simulink model "Digital-Memory-Architecture"  (R2024b)
settings: Solver=VariableStepAuto  StartTime=0.0  StopTime=10.0  RelTol=1e-3
libraries: simulink_extras x129
(part 3 of 5)

== system Digital-Memory-Architecture/BitCell23 ==
  D : Inport
  WE : Inport  Port=2
  CLK : Inport  Port=3
  Constant : Constant
  D Flip-Flop : simulink_extras/Flip Flops/D Flip-Flop
  Logical Operator : Logic  Operator=NOT  IconShape=distinctive  AllPortsSameDT=off  OutDataTypeStr=boolean
  Logical Operator1 : Logic  IconShape=distinctive  AllPortsSameDT=off  OutDataTypeStr=boolean
  Logical Operator2 : Logic  IconShape=distinctive  AllPortsSameDT=off  OutDataTypeStr=boolean
  Logical Operator3 : Logic  Operator=OR  IconShape=distinctive  AllPortsSameDT=off  OutDataTypeStr=boolean
  Q : Outport
  wires:
  Logical Operator2/1 -> Logical Operator3/2
  CLK/1 -> D Flip-Flop/2
  Logical Operator1/1 -> Logical Operator3/1
  Constant/1 -> D Flip-Flop/3
  D Flip-Flop/1 -> Q/1, Logical Operator2/2
  Logical Operator3/1 -> D Flip-Flop/1
  Logical Operator/1 -> Logical Operator2/1
  WE/1 -> Logical Operator/1, Logical Operator1/2
  D/1 -> Logical Operator1/1

== system Digital-Memory-Architecture/BitCell24 ==
  D : Inport
  WE : Inport  Port=2
  CLK : Inport  Port=3
  Constant : Constant
  D Flip-Flop : simulink_extras/Flip Flops/D Flip-Flop
  Logical Operator : Logic  Operator=NOT  IconShape=distinctive  AllPortsSameDT=off  OutDataTypeStr=boolean
  Logical Operator1 : Logic  IconShape=distinctive  AllPortsSameDT=off  OutDataTypeStr=boolean
  Logical Operator2 : Logic  IconShape=distinctive  AllPortsSameDT=off  OutDataTypeStr=boolean
  Logical Operator3 : Logic  Operator=OR  IconShape=distinctive  AllPortsSameDT=off  OutDataTypeStr=boolean
  Q : Outport
  wires:
  Logical Operator2/1 -> Logical Operator3/2
  CLK/1 -> D Flip-Flop/2
  Logical Operator1/1 -> Logical Operator3/1
  Constant/1 -> D Flip-Flop/3
  D Flip-Flop/1 -> Q/1, Logical Operator2/2
  Logical Operator3/1 -> D Flip-Flop/1
  Logical Operator/1 -> Logical Operator2/1
  WE/1 -> Logical Operator/1, Logical Operator1/2
  D/1 -> Logical Operator1/1

== system Digital-Memory-Architecture/BitCell25 ==
  D : Inport
  WE : Inport  Port=2
  CLK : Inport  Port=3
  Constant : Constant
  D Flip-Flop : simulink_extras/Flip Flops/D Flip-Flop
  Logical Operator : Logic  Operator=NOT  IconShape=distinctive  AllPortsSameDT=off  OutDataTypeStr=boolean
  Logical Operator1 : Logic  IconShape=distinctive  AllPortsSameDT=off  OutDataTypeStr=boolean
  Logical Operator2 : Logic  IconShape=distinctive  AllPortsSameDT=off  OutDataTypeStr=boolean
  Logical Operator3 : Logic  Operator=OR  IconShape=distinctive  AllPortsSameDT=off  OutDataTypeStr=boolean
  Q : Outport
  wires:
  Logical Operator2/1 -> Logical Operator3/2
  CLK/1 -> D Flip-Flop/2
  Logical Operator1/1 -> Logical Operator3/1
  Constant/1 -> D Flip-Flop/3
  D Flip-Flop/1 -> Q/1, Logical Operator2/2
  Logical Operator3/1 -> D Flip-Flop/1
  Logical Operator/1 -> Logical Operator2/1
  WE/1 -> Logical Operator/1, Logical Operator1/2
  D/1 -> Logical Operator1/1

== system Digital-Memory-Architecture/BitCell26 ==
  D : Inport
  WE : Inport  Port=2
  CLK : Inport  Port=3
  Constant : Constant
  D Flip-Flop : simulink_extras/Flip Flops/D Flip-Flop
  Logical Operator : Logic  Operator=NOT  IconShape=distinctive  AllPortsSameDT=off  OutDataTypeStr=boolean
  Logical Operator1 : Logic  IconShape=distinctive  AllPortsSameDT=off  OutDataTypeStr=boolean
  Logical Operator2 : Logic  IconShape=distinctive  AllPortsSameDT=off  OutDataTypeStr=boolean
  Logical Operator3 : Logic  Operator=OR  IconShape=distinctive  AllPortsSameDT=off  OutDataTypeStr=boolean
  Q : Outport
  wires:
  Logical Operator2/1 -> Logical Operator3/2
  CLK/1 -> D Flip-Flop/2
  Logical Operator1/1 -> Logical Operator3/1
  Constant/1 -> D Flip-Flop/3
  D Flip-Flop/1 -> Q/1, Logical Operator2/2
  Logical Operator3/1 -> D Flip-Flop/1
  Logical Operator/1 -> Logical Operator2/1
  WE/1 -> Logical Operator/1, Logical Operator1/2
  D/1 -> Logical Operator1/1

== system Digital-Memory-Architecture/BitCell27 ==
  D : Inport
  WE : Inport  Port=2
  CLK : Inport  Port=3
  Constant : Constant
  D Flip-Flop : simulink_extras/Flip Flops/D Flip-Flop
  Logical Operator : Logic  Operator=NOT  IconShape=distinctive  AllPortsSameDT=off  OutDataTypeStr=boolean
  Logical Operator1 : Logic  IconShape=distinctive  AllPortsSameDT=off  OutDataTypeStr=boolean
  Logical Operator2 : Logic  IconShape=distinctive  AllPortsSameDT=off  OutDataTypeStr=boolean
  Logical Operator3 : Logic  Operator=OR  IconShape=distinctive  AllPortsSameDT=off  OutDataTypeStr=boolean
  Q : Outport
  wires:
  Logical Operator2/1 -> Logical Operator3/2
  CLK/1 -> D Flip-Flop/2
  Logical Operator1/1 -> Logical Operator3/1
  Constant/1 -> D Flip-Flop/3
  D Flip-Flop/1 -> Q/1, Logical Operator2/2
  Logical Operator3/1 -> D Flip-Flop/1
  Logical Operator/1 -> Logical Operator2/1
  WE/1 -> Logical Operator/1, Logical Operator1/2
  D/1 -> Logical Operator1/1

== system Digital-Memory-Architecture/BitCell28 ==
  D : Inport
  WE : Inport  Port=2
  CLK : Inport  Port=3
  Constant : Constant
  D Flip-Flop : simulink_extras/Flip Flops/D Flip-Flop
  Logical Operator : Logic  Operator=NOT  IconShape=distinctive  AllPortsSameDT=off  OutDataTypeStr=boolean
  Logical Operator1 : Logic  IconShape=distinctive  AllPortsSameDT=off  OutDataTypeStr=boolean
  Logical Operator2 : Logic  IconShape=distinctive  AllPortsSameDT=off  OutDataTypeStr=boolean
  Logical Operator3 : Logic  Operator=OR  IconShape=distinctive  AllPortsSameDT=off  OutDataTypeStr=boolean
  Q : Outport
  wires:
  Logical Operator2/1 -> Logical Operator3/2
  CLK/1 -> D Flip-Flop/2
  Logical Operator1/1 -> Logical Operator3/1
  Constant/1 -> D Flip-Flop/3
  D Flip-Flop/1 -> Q/1, Logical Operator2/2
  Logical Operator3/1 -> D Flip-Flop/1
  Logical Operator/1 -> Logical Operator2/1
  WE/1 -> Logical Operator/1, Logical Operator1/2
  D/1 -> Logical Operator1/1

== system Digital-Memory-Architecture/BitCell29 ==
  D : Inport
  WE : Inport  Port=2
  CLK : Inport  Port=3
  Constant : Constant
  D Flip-Flop : simulink_extras/Flip Flops/D Flip-Flop
  Logical Operator : Logic  Operator=NOT  IconShape=distinctive  AllPortsSameDT=off  OutDataTypeStr=boolean
  Logical Operator1 : Logic  IconShape=distinctive  AllPortsSameDT=off  OutDataTypeStr=boolean
  Logical Operator2 : Logic  IconShape=distinctive  AllPortsSameDT=off  OutDataTypeStr=boolean
  Logical Operator3 : Logic  Operator=OR  IconShape=distinctive  AllPortsSameDT=off  OutDataTypeStr=boolean
  Q : Outport
  wires:
  Logical Operator2/1 -> Logical Operator3/2
  CLK/1 -> D Flip-Flop/2
  Logical Operator1/1 -> Logical Operator3/1
  Constant/1 -> D Flip-Flop/3
  D Flip-Flop/1 -> Q/1, Logical Operator2/2
  Logical Operator3/1 -> D Flip-Flop/1
  Logical Operator/1 -> Logical Operator2/1
  WE/1 -> Logical Operator/1, Logical Operator1/2
  D/1 -> Logical Operator1/1

== system Digital-Memory-Architecture/BitCell3 ==
  D : Inport
  WE : Inport  Port=2
  CLK : Inport  Port=3
  Constant : Constant
  D Flip-Flop : simulink_extras/Flip Flops/D Flip-Flop
  Logical Operator : Logic  Operator=NOT  IconShape=distinctive  AllPortsSameDT=off  OutDataTypeStr=boolean
  Logical Operator1 : Logic  IconShape=distinctive  AllPortsSameDT=off  OutDataTypeStr=boolean
  Logical Operator2 : Logic  IconShape=distinctive  AllPortsSameDT=off  OutDataTypeStr=boolean
  Logical Operator3 : Logic  Operator=OR  IconShape=distinctive  AllPortsSameDT=off  OutDataTypeStr=boolean
  Q : Outport
  wires:
  Logical Operator2/1 -> Logical Operator3/2
  CLK/1 -> D Flip-Flop/2
  Logical Operator1/1 -> Logical Operator3/1
  Constant/1 -> D Flip-Flop/3
  D Flip-Flop/1 -> Q/1, Logical Operator2/2
  Logical Operator3/1 -> D Flip-Flop/1
  Logical Operator/1 -> Logical Operator2/1
  WE/1 -> Logical Operator/1, Logical Operator1/2
  D/1 -> Logical Operator1/1

== system Digital-Memory-Architecture/BitCell30 ==
  D : Inport
  WE : Inport  Port=2
  CLK : Inport  Port=3
  Constant : Constant
  D Flip-Flop : simulink_extras/Flip Flops/D Flip-Flop
  Logical Operator : Logic  Operator=NOT  IconShape=distinctive  AllPortsSameDT=off  OutDataTypeStr=boolean
  Logical Operator1 : Logic  IconShape=distinctive  AllPortsSameDT=off  OutDataTypeStr=boolean
  Logical Operator2 : Logic  IconShape=distinctive  AllPortsSameDT=off  OutDataTypeStr=boolean
  Logical Operator3 : Logic  Operator=OR  IconShape=distinctive  AllPortsSameDT=off  OutDataTypeStr=boolean
  Q : Outport
  wires:
  Logical Operator2/1 -> Logical Operator3/2
  CLK/1 -> D Flip-Flop/2
  Logical Operator1/1 -> Logical Operator3/1
  Constant/1 -> D Flip-Flop/3
  D Flip-Flop/1 -> Q/1, Logical Operator2/2
  Logical Operator3/1 -> D Flip-Flop/1
  Logical Operator/1 -> Logical Operator2/1
  WE/1 -> Logical Operator/1, Logical Operator1/2
  D/1 -> Logical Operator1/1

== system Digital-Memory-Architecture/BitCell31 ==
  D : Inport
  WE : Inport  Port=2
  CLK : Inport  Port=3
  Constant : Constant
  D Flip-Flop : simulink_extras/Flip Flops/D Flip-Flop
  Logical Operator : Logic  Operator=NOT  IconShape=distinctive  AllPortsSameDT=off  OutDataTypeStr=boolean
  Logical Operator1 : Logic  IconShape=distinctive  AllPortsSameDT=off  OutDataTypeStr=boolean
  Logical Operator2 : Logic  IconShape=distinctive  AllPortsSameDT=off  OutDataTypeStr=boolean
  Logical Operator3 : Logic  Operator=OR  IconShape=distinctive  AllPortsSameDT=off  OutDataTypeStr=boolean
  Q : Outport
  wires:
  Logical Operator2/1 -> Logical Operator3/2
  CLK/1 -> D Flip-Flop/2
  Logical Operator1/1 -> Logical Operator3/1
  Constant/1 -> D Flip-Flop/3
  D Flip-Flop/1 -> Q/1, Logical Operator2/2
  Logical Operator3/1 -> D Flip-Flop/1
  Logical Operator/1 -> Logical Operator2/1
  WE/1 -> Logical Operator/1, Logical Operator1/2
  D/1 -> Logical Operator1/1

== system Digital-Memory-Architecture/BitCell32 ==
  D : Inport
  WE : Inport  Port=2
  CLK : Inport  Port=3
  Constant : Constant
  D Flip-Flop : simulink_extras/Flip Flops/D Flip-Flop
  Logical Operator : Logic  Operator=NOT  IconShape=distinctive  AllPortsSameDT=off  OutDataTypeStr=boolean
  Logical Operator1 : Logic  IconShape=distinctive  AllPortsSameDT=off  OutDataTypeStr=boolean
  Logical Operator2 : Logic  IconShape=distinctive  AllPortsSameDT=off  OutDataTypeStr=boolean
  Logical Operator3 : Logic  Operator=OR  IconShape=distinctive  AllPortsSameDT=off  OutDataTypeStr=boolean
  Q : Outport
  wires:
  Logical Operator2/1 -> Logical Operator3/2
  CLK/1 -> D Flip-Flop/2
  Logical Operator1/1 -> Logical Operator3/1
  Constant/1 -> D Flip-Flop/3
  D Flip-Flop/1 -> Q/1, Logical Operator2/2
  Logical Operator3/1 -> D Flip-Flop/1
  Logical Operator/1 -> Logical Operator2/1
  WE/1 -> Logical Operator/1, Logical Operator1/2
  D/1 -> Logical Operator1/1

== system Digital-Memory-Architecture/BitCell33 ==
  D : Inport
  WE : Inport  Port=2
  CLK : Inport  Port=3
  Constant : Constant
  D Flip-Flop : simulink_extras/Flip Flops/D Flip-Flop
  Logical Operator : Logic  Operator=NOT  IconShape=distinctive  AllPortsSameDT=off  OutDataTypeStr=boolean
  Logical Operator1 : Logic  IconShape=distinctive  AllPortsSameDT=off  OutDataTypeStr=boolean
  Logical Operator2 : Logic  IconShape=distinctive  AllPortsSameDT=off  OutDataTypeStr=boolean
  Logical Operator3 : Logic  Operator=OR  IconShape=distinctive  AllPortsSameDT=off  OutDataTypeStr=boolean
  Q : Outport
  wires:
  Logical Operator2/1 -> Logical Operator3/2
  CLK/1 -> D Flip-Flop/2
  Logical Operator1/1 -> Logical Operator3/1
  Constant/1 -> D Flip-Flop/3
  D Flip-Flop/1 -> Q/1, Logical Operator2/2
  Logical Operator3/1 -> D Flip-Flop/1
  Logical Operator/1 -> Logical Operator2/1
  WE/1 -> Logical Operator/1, Logical Operator1/2
  D/1 -> Logical Operator1/1

== system Digital-Memory-Architecture/BitCell34 ==
  D : Inport
  WE : Inport  Port=2
  CLK : Inport  Port=3
  Constant : Constant
  D Flip-Flop : simulink_extras/Flip Flops/D Flip-Flop
  Logical Operator : Logic  Operator=NOT  IconShape=distinctive  AllPortsSameDT=off  OutDataTypeStr=boolean
  Logical Operator1 : Logic  IconShape=distinctive  AllPortsSameDT=off  OutDataTypeStr=boolean
  Logical Operator2 : Logic  IconShape=distinctive  AllPortsSameDT=off  OutDataTypeStr=boolean
  Logical Operator3 : Logic  Operator=OR  IconShape=distinctive  AllPortsSameDT=off  OutDataTypeStr=boolean
  Q : Outport
  wires:
  Logical Operator2/1 -> Logical Operator3/2
  CLK/1 -> D Flip-Flop/2
  Logical Operator1/1 -> Logical Operator3/1
  Constant/1 -> D Flip-Flop/3
  D Flip-Flop/1 -> Q/1, Logical Operator2/2
  Logical Operator3/1 -> D Flip-Flop/1
  Logical Operator/1 -> Logical Operator2/1
  WE/1 -> Logical Operator/1, Logical Operator1/2
  D/1 -> Logical Operator1/1

== system Digital-Memory-Architecture/BitCell35 ==
  D : Inport
  WE : Inport  Port=2
  CLK : Inport  Port=3
  Constant : Constant
  D Flip-Flop : simulink_extras/Flip Flops/D Flip-Flop
  Logical Operator : Logic  Operator=NOT  IconShape=distinctive  AllPortsSameDT=off  OutDataTypeStr=boolean
  Logical Operator1 : Logic  IconShape=distinctive  AllPortsSameDT=off  OutDataTypeStr=boolean
  Logical Operator2 : Logic  IconShape=distinctive  AllPortsSameDT=off  OutDataTypeStr=boolean
  Logical Operator3 : Logic  Operator=OR  IconShape=distinctive  AllPortsSameDT=off  OutDataTypeStr=boolean
  Q : Outport
  wires:
  Logical Operator2/1 -> Logical Operator3/2
  CLK/1 -> D Flip-Flop/2
  Logical Operator1/1 -> Logical Operator3/1
  Constant/1 -> D Flip-Flop/3
  D Flip-Flop/1 -> Q/1, Logical Operator2/2
  Logical Operator3/1 -> D Flip-Flop/1
  Logical Operator/1 -> Logical Operator2/1
  WE/1 -> Logical Operator/1, Logical Operator1/2
  D/1 -> Logical Operator1/1

== system Digital-Memory-Architecture/BitCell36 ==
  D : Inport
  WE : Inport  Port=2
  CLK : Inport  Port=3
  Constant : Constant
  D Flip-Flop : simulink_extras/Flip Flops/D Flip-Flop
  Logical Operator : Logic  Operator=NOT  IconShape=distinctive  AllPortsSameDT=off  OutDataTypeStr=boolean
  Logical Operator1 : Logic  IconShape=distinctive  AllPortsSameDT=off  OutDataTypeStr=boolean
  Logical Operator2 : Logic  IconShape=distinctive  AllPortsSameDT=off  OutDataTypeStr=boolean
  Logical Operator3 : Logic  Operator=OR  IconShape=distinctive  AllPortsSameDT=off  OutDataTypeStr=boolean
  Q : Outport
  wires:
  Logical Operator2/1 -> Logical Operator3/2
  CLK/1 -> D Flip-Flop/2
  Logical Operator1/1 -> Logical Operator3/1
  Constant/1 -> D Flip-Flop/3
  D Flip-Flop/1 -> Q/1, Logical Operator2/2
  Logical Operator3/1 -> D Flip-Flop/1
  Logical Operator/1 -> Logical Operator2/1
  WE/1 -> Logical Operator/1, Logical Operator1/2
  D/1 -> Logical Operator1/1

== system Digital-Memory-Architecture/BitCell37 ==
  D : Inport
  WE : Inport  Port=2
  CLK : Inport  Port=3
  Constant : Constant
  D Flip-Flop : simulink_extras/Flip Flops/D Flip-Flop
  Logical Operator : Logic  Operator=NOT  IconShape=distinctive  AllPortsSameDT=off  OutDataTypeStr=boolean
  Logical Operator1 : Logic  IconShape=distinctive  AllPortsSameDT=off  OutDataTypeStr=boolean
  Logical Operator2 : Logic  IconShape=distinctive  AllPortsSameDT=off  OutDataTypeStr=boolean
  Logical Operator3 : Logic  Operator=OR  IconShape=distinctive  AllPortsSameDT=off  OutDataTypeStr=boolean
  Q : Outport
  wires:
  Logical Operator2/1 -> Logical Operator3/2
  CLK/1 -> D Flip-Flop/2
  Logical Operator1/1 -> Logical Operator3/1
  Constant/1 -> D Flip-Flop/3
  D Flip-Flop/1 -> Q/1, Logical Operator2/2
  Logical Operator3/1 -> D Flip-Flop/1
  Logical Operator/1 -> Logical Operator2/1
  WE/1 -> Logical Operator/1, Logical Operator1/2
  D/1 -> Logical Operator1/1

== system Digital-Memory-Architecture/BitCell38 ==
  D : Inport
  WE : Inport  Port=2
  CLK : Inport  Port=3
  Constant : Constant
  D Flip-Flop : simulink_extras/Flip Flops/D Flip-Flop
  Logical Operator : Logic  Operator=NOT  IconShape=distinctive  AllPortsSameDT=off  OutDataTypeStr=boolean
  Logical Operator1 : Logic  IconShape=distinctive  AllPortsSameDT=off  OutDataTypeStr=boolean
  Logical Operator2 : Logic  IconShape=distinctive  AllPortsSameDT=off  OutDataTypeStr=boolean
  Logical Operator3 : Logic  Operator=OR  IconShape=distinctive  AllPortsSameDT=off  OutDataTypeStr=boolean
  Q : Outport
  wires:
  Logical Operator2/1 -> Logical Operator3/2
  CLK/1 -> D Flip-Flop/2
  Logical Operator1/1 -> Logical Operator3/1
  Constant/1 -> D Flip-Flop/3
  D Flip-Flop/1 -> Q/1, Logical Operator2/2
  Logical Operator3/1 -> D Flip-Flop/1
  Logical Operator/1 -> Logical Operator2/1
  WE/1 -> Logical Operator/1, Logical Operator1/2
  D/1 -> Logical Operator1/1

== system Digital-Memory-Architecture/BitCell39 ==
  D : Inport
  WE : Inport  Port=2
  CLK : Inport  Port=3
  Constant : Constant
  D Flip-Flop : simulink_extras/Flip Flops/D Flip-Flop
  Logical Operator : Logic  Operator=NOT  IconShape=distinctive  AllPortsSameDT=off  OutDataTypeStr=boolean
  Logical Operator1 : Logic  IconShape=distinctive  AllPortsSameDT=off  OutDataTypeStr=boolean
  Logical Operator2 : Logic  IconShape=distinctive  AllPortsSameDT=off  OutDataTypeStr=boolean
  Logical Operator3 : Logic  Operator=OR  IconShape=distinctive  AllPortsSameDT=off  OutDataTypeStr=boolean
  Q : Outport
  wires:
  Logical Operator2/1 -> Logical Operator3/2
  CLK/1 -> D Flip-Flop/2
  Logical Operator1/1 -> Logical Operator3/1
  Constant/1 -> D Flip-Flop/3
  D Flip-Flop/1 -> Q/1, Logical Operator2/2
  Logical Operator3/1 -> D Flip-Flop/1
  Logical Operator/1 -> Logical Operator2/1
  WE/1 -> Logical Operator/1, Logical Operator1/2
  D/1 -> Logical Operator1/1

== system Digital-Memory-Architecture/BitCell4 ==
  D : Inport
  WE : Inport  Port=2
  CLK : Inport  Port=3
  Constant : Constant
  D Flip-Flop : simulink_extras/Flip Flops/D Flip-Flop
  Logical Operator : Logic  Operator=NOT  IconShape=distinctive  AllPortsSameDT=off  OutDataTypeStr=boolean
  Logical Operator1 : Logic  IconShape=distinctive  AllPortsSameDT=off  OutDataTypeStr=boolean
  Logical Operator2 : Logic  IconShape=distinctive  AllPortsSameDT=off  OutDataTypeStr=boolean
  Logical Operator3 : Logic  Operator=OR  IconShape=distinctive  AllPortsSameDT=off  OutDataTypeStr=boolean
  Q : Outport
  wires:
  Logical Operator2/1 -> Logical Operator3/2
  CLK/1 -> D Flip-Flop/2
  Logical Operator1/1 -> Logical Operator3/1
  Constant/1 -> D Flip-Flop/3
  D Flip-Flop/1 -> Q/1, Logical Operator2/2
  Logical Operator3/1 -> D Flip-Flop/1
  Logical Operator/1 -> Logical Operator2/1
  WE/1 -> Logical Operator/1, Logical Operator1/2
  D/1 -> Logical Operator1/1

== system Digital-Memory-Architecture/BitCell40 ==
  D : Inport
  WE : Inport  Port=2
  CLK : Inport  Port=3
  Constant : Constant
  D Flip-Flop : simulink_extras/Flip Flops/D Flip-Flop
  Logical Operator : Logic  Operator=NOT  IconShape=distinctive  AllPortsSameDT=off  OutDataTypeStr=boolean
  Logical Operator1 : Logic  IconShape=distinctive  AllPortsSameDT=off  OutDataTypeStr=boolean
  Logical Operator2 : Logic  IconShape=distinctive  AllPortsSameDT=off  OutDataTypeStr=boolean
  Logical Operator3 : Logic  Operator=OR  IconShape=distinctive  AllPortsSameDT=off  OutDataTypeStr=boolean
  Q : Outport
  wires:
  Logical Operator2/1 -> Logical Operator3/2
  CLK/1 -> D Flip-Flop/2
  Logical Operator1/1 -> Logical Operator3/1
  Constant/1 -> D Flip-Flop/3
  D Flip-Flop/1 -> Q/1, Logical Operator2/2
  Logical Operator3/1 -> D Flip-Flop/1
  Logical Operator/1 -> Logical Operator2/1
  WE/1 -> Logical Operator/1, Logical Operator1/2
  D/1 -> Logical Operator1/1

== system Digital-Memory-Architecture/BitCell41 ==
  D : Inport
  WE : Inport  Port=2
  CLK : Inport  Port=3
  Constant : Constant
  D Flip-Flop : simulink_extras/Flip Flops/D Flip-Flop
  Logical Operator : Logic  Operator=NOT  IconShape=distinctive  AllPortsSameDT=off  OutDataTypeStr=boolean
  Logical Operator1 : Logic  IconShape=distinctive  AllPortsSameDT=off  OutDataTypeStr=boolean
  Logical Operator2 : Logic  IconShape=distinctive  AllPortsSameDT=off  OutDataTypeStr=boolean
  Logical Operator3 : Logic  Operator=OR  IconShape=distinctive  AllPortsSameDT=off  OutDataTypeStr=boolean
  Q : Outport
  wires:
  Logical Operator2/1 -> Logical Operator3/2
  CLK/1 -> D Flip-Flop/2
  Logical Operator1/1 -> Logical Operator3/1
  Constant/1 -> D Flip-Flop/3
  D Flip-Flop/1 -> Q/1, Logical Operator2/2
  Logical Operator3/1 -> D Flip-Flop/1
  Logical Operator/1 -> Logical Operator2/1
  WE/1 -> Logical Operator/1, Logical Operator1/2
  D/1 -> Logical Operator1/1

== system Digital-Memory-Architecture/BitCell42 ==
  D : Inport
  WE : Inport  Port=2
  CLK : Inport  Port=3
  Constant : Constant
  D Flip-Flop : simulink_extras/Flip Flops/D Flip-Flop
  Logical Operator : Logic  Operator=NOT  IconShape=distinctive  AllPortsSameDT=off  OutDataTypeStr=boolean
  Logical Operator1 : Logic  IconShape=distinctive  AllPortsSameDT=off  OutDataTypeStr=boolean
  Logical Operator2 : Logic  IconShape=distinctive  AllPortsSameDT=off  OutDataTypeStr=boolean
  Logical Operator3 : Logic  Operator=OR  IconShape=distinctive  AllPortsSameDT=off  OutDataTypeStr=boolean
  Q : Outport
  wires:
  Logical Operator2/1 -> Logical Operator3/2
  CLK/1 -> D Flip-Flop/2
  Logical Operator1/1 -> Logical Operator3/1
  Constant/1 -> D Flip-Flop/3
  D Flip-Flop/1 -> Q/1, Logical Operator2/2
  Logical Operator3/1 -> D Flip-Flop/1
  Logical Operator/1 -> Logical Operator2/1
  WE/1 -> Logical Operator/1, Logical Operator1/2
  D/1 -> Logical Operator1/1

== system Digital-Memory-Architecture/BitCell43 ==
  D : Inport
  WE : Inport  Port=2
  CLK : Inport  Port=3
  Constant : Constant
  D Flip-Flop : simulink_extras/Flip Flops/D Flip-Flop
  Logical Operator : Logic  Operator=NOT  IconShape=distinctive  AllPortsSameDT=off  OutDataTypeStr=boolean
  Logical Operator1 : Logic  IconShape=distinctive  AllPortsSameDT=off  OutDataTypeStr=boolean
  Logical Operator2 : Logic  IconShape=distinctive  AllPortsSameDT=off  OutDataTypeStr=boolean
  Logical Operator3 : Logic  Operator=OR  IconShape=distinctive  AllPortsSameDT=off  OutDataTypeStr=boolean
  Q : Outport
  wires:
  Logical Operator2/1 -> Logical Operator3/2
  CLK/1 -> D Flip-Flop/2
  Logical Operator1/1 -> Logical Operator3/1
  Constant/1 -> D Flip-Flop/3
  D Flip-Flop/1 -> Q/1, Logical Operator2/2
  Logical Operator3/1 -> D Flip-Flop/1
  Logical Operator/1 -> Logical Operator2/1
  WE/1 -> Logical Operator/1, Logical Operator1/2
  D/1 -> Logical Operator1/1

== system Digital-Memory-Architecture/BitCell44 ==
  D : Inport
  WE : Inport  Port=2
  CLK : Inport  Port=3
  Constant : Constant
  D Flip-Flop : simulink_extras/Flip Flops/D Flip-Flop
  Logical Operator : Logic  Operator=NOT  IconShape=distinctive  AllPortsSameDT=off  OutDataTypeStr=boolean
  Logical Operator1 : Logic  IconShape=distinctive  AllPortsSameDT=off  OutDataTypeStr=boolean
  Logical Operator2 : Logic  IconShape=distinctive  AllPortsSameDT=off  OutDataTypeStr=boolean
  Logical Operator3 : Logic  Operator=OR  IconShape=distinctive  AllPortsSameDT=off  OutDataTypeStr=boolean
  Q : Outport
  wires:
  Logical Operator2/1 -> Logical Operator3/2
  CLK/1 -> D Flip-Flop/2
  Logical Operator1/1 -> Logical Operator3/1
  Constant/1 -> D Flip-Flop/3
  D Flip-Flop/1 -> Q/1, Logical Operator2/2
  Logical Operator3/1 -> D Flip-Flop/1
  Logical Operator/1 -> Logical Operator2/1
  WE/1 -> Logical Operator/1, Logical Operator1/2
  D/1 -> Logical Operator1/1

== system Digital-Memory-Architecture/BitCell45 ==
  D : Inport
  WE : Inport  Port=2
  CLK : Inport  Port=3
  Constant : Constant
  D Flip-Flop : simulink_extras/Flip Flops/D Flip-Flop
  Logical Operator : Logic  Operator=NOT  IconShape=distinctive  AllPortsSameDT=off  OutDataTypeStr=boolean
  Logical Operator1 : Logic  IconShape=distinctive  AllPortsSameDT=off  OutDataTypeStr=boolean
  Logical Operator2 : Logic  IconShape=distinctive  AllPortsSameDT=off  OutDataTypeStr=boolean
  Logical Operator3 : Logic  Operator=OR  IconShape=distinctive  AllPortsSameDT=off  OutDataTypeStr=boolean
  Q : Outport
  wires:
  Logical Operator2/1 -> Logical Operator3/2
  CLK/1 -> D Flip-Flop/2
  Logical Operator1/1 -> Logical Operator3/1
  Constant/1 -> D Flip-Flop/3
  D Flip-Flop/1 -> Q/1, Logical Operator2/2
  Logical Operator3/1 -> D Flip-Flop/1
  Logical Operator/1 -> Logical Operator2/1
  WE/1 -> Logical Operator/1, Logical Operator1/2
  D/1 -> Logical Operator1/1

== system Digital-Memory-Architecture/BitCell46 ==
  D : Inport
  WE : Inport  Port=2
  CLK : Inport  Port=3
  Constant : Constant
  D Flip-Flop : simulink_extras/Flip Flops/D Flip-Flop
  Logical Operator : Logic  Operator=NOT  IconShape=distinctive  AllPortsSameDT=off  OutDataTypeStr=boolean
  Logical Operator1 : Logic  IconShape=distinctive  AllPortsSameDT=off  OutDataTypeStr=boolean
  Logical Operator2 : Logic  IconShape=distinctive  AllPortsSameDT=off  OutDataTypeStr=boolean
  Logical Operator3 : Logic  Operator=OR  IconShape=distinctive  AllPortsSameDT=off  OutDataTypeStr=boolean
  Q : Outport
  wires:
  Logical Operator2/1 -> Logical Operator3/2
  CLK/1 -> D Flip-Flop/2
  Logical Operator1/1 -> Logical Operator3/1
  Constant/1 -> D Flip-Flop/3
  D Flip-Flop/1 -> Q/1, Logical Operator2/2
  Logical Operator3/1 -> D Flip-Flop/1
  Logical Operator/1 -> Logical Operator2/1
  WE/1 -> Logical Operator/1, Logical Operator1/2
  D/1 -> Logical Operator1/1

== system Digital-Memory-Architecture/BitCell47 ==
  D : Inport
  WE : Inport  Port=2
  CLK : Inport  Port=3
  Constant : Constant
  D Flip-Flop : simulink_extras/Flip Flops/D Flip-Flop
  Logical Operator : Logic  Operator=NOT  IconShape=distinctive  AllPortsSameDT=off  OutDataTypeStr=boolean
  Logical Operator1 : Logic  IconShape=distinctive  AllPortsSameDT=off  OutDataTypeStr=boolean
  Logical Operator2 : Logic  IconShape=distinctive  AllPortsSameDT=off  OutDataTypeStr=boolean
  Logical Operator3 : Logic  Operator=OR  IconShape=distinctive  AllPortsSameDT=off  OutDataTypeStr=boolean
  Q : Outport
  wires:
  Logical Operator2/1 -> Logical Operator3/2
  CLK/1 -> D Flip-Flop/2
  Logical Operator1/1 -> Logical Operator3/1
  Constant/1 -> D Flip-Flop/3
  D Flip-Flop/1 -> Q/1, Logical Operator2/2
  Logical Operator3/1 -> D Flip-Flop/1
  Logical Operator/1 -> Logical Operator2/1
  WE/1 -> Logical Operator/1, Logical Operator1/2
  D/1 -> Logical Operator1/1

== system Digital-Memory-Architecture/BitCell48 ==
  D : Inport
  WE : Inport  Port=2
  CLK : Inport  Port=3
  Constant : Constant
  D Flip-Flop : simulink_extras/Flip Flops/D Flip-Flop
  Logical Operator : Logic  Operator=NOT  IconShape=distinctive  AllPortsSameDT=off  OutDataTypeStr=boolean
  Logical Operator1 : Logic  IconShape=distinctive  AllPortsSameDT=off  OutDataTypeStr=boolean
  Logical Operator2 : Logic  IconShape=distinctive  AllPortsSameDT=off  OutDataTypeStr=boolean
  Logical Operator3 : Logic  Operator=OR  IconShape=distinctive  AllPortsSameDT=off  OutDataTypeStr=boolean
  Q : Outport
  wires:
  Logical Operator2/1 -> Logical Operator3/2
  CLK/1 -> D Flip-Flop/2
  Logical Operator1/1 -> Logical Operator3/1
  Constant/1 -> D Flip-Flop/3
  D Flip-Flop/1 -> Q/1, Logical Operator2/2
  Logical Operator3/1 -> D Flip-Flop/1
  Logical Operator/1 -> Logical Operator2/1
  WE/1 -> Logical Operator/1, Logical Operator1/2
  D/1 -> Logical Operator1/1

== system Digital-Memory-Architecture/BitCell49 ==
  D : Inport
  WE : Inport  Port=2
  CLK : Inport  Port=3
  Constant : Constant
  D Flip-Flop : simulink_extras/Flip Flops/D Flip-Flop
  Logical Operator : Logic  Operator=NOT  IconShape=distinctive  AllPortsSameDT=off  OutDataTypeStr=boolean
  Logical Operator1 : Logic  IconShape=distinctive  AllPortsSameDT=off  OutDataTypeStr=boolean
  Logical Operator2 : Logic  IconShape=distinctive  AllPortsSameDT=off  OutDataTypeStr=boolean
  Logical Operator3 : Logic  Operator=OR  IconShape=distinctive  AllPortsSameDT=off  OutDataTypeStr=boolean
  Q : Outport
  wires:
  Logical Operator2/1 -> Logical Operator3/2
  CLK/1 -> D Flip-Flop/2
  Logical Operator1/1 -> Logical Operator3/1
  Constant/1 -> D Flip-Flop/3
  D Flip-Flop/1 -> Q/1, Logical Operator2/2
  Logical Operator3/1 -> D Flip-Flop/1
  Logical Operator/1 -> Logical Operator2/1
  WE/1 -> Logical Operator/1, Logical Operator1/2
  D/1 -> Logical Operator1/1

== system Digital-Memory-Architecture/BitCell5 ==
  D : Inport
  WE : Inport  Port=2
  CLK : Inport  Port=3
  Constant : Constant
  D Flip-Flop : simulink_extras/Flip Flops/D Flip-Flop
  Logical Operator : Logic  Operator=NOT  IconShape=distinctive  AllPortsSameDT=off  OutDataTypeStr=boolean
  Logical Operator1 : Logic  IconShape=distinctive  AllPortsSameDT=off  OutDataTypeStr=boolean
  Logical Operator2 : Logic  IconShape=distinctive  AllPortsSameDT=off  OutDataTypeStr=boolean
  Logical Operator3 : Logic  Operator=OR  IconShape=distinctive  AllPortsSameDT=off  OutDataTypeStr=boolean
  Q : Outport
  wires:
  Logical Operator2/1 -> Logical Operator3/2
  CLK/1 -> D Flip-Flop/2
  Logical Operator1/1 -> Logical Operator3/1
  Constant/1 -> D Flip-Flop/3
  D Flip-Flop/1 -> Q/1, Logical Operator2/2
  Logical Operator3/1 -> D Flip-Flop/1
  Logical Operator/1 -> Logical Operator2/1
  WE/1 -> Logical Operator/1, Logical Operator1/2
  D/1 -> Logical Operator1/1

== system Digital-Memory-Architecture/BitCell50 ==
  D : Inport
  WE : Inport  Port=2
  CLK : Inport  Port=3
  Constant : Constant
  D Flip-Flop : simulink_extras/Flip Flops/D Flip-Flop
  Logical Operator : Logic  Operator=NOT  IconShape=distinctive  AllPortsSameDT=off  OutDataTypeStr=boolean
  Logical Operator1 : Logic  IconShape=distinctive  AllPortsSameDT=off  OutDataTypeStr=boolean
  Logical Operator2 : Logic  IconShape=distinctive  AllPortsSameDT=off  OutDataTypeStr=boolean
  Logical Operator3 : Logic  Operator=OR  IconShape=distinctive  AllPortsSameDT=off  OutDataTypeStr=boolean
  Q : Outport
  wires:
  Logical Operator2/1 -> Logical Operator3/2
  CLK/1 -> D Flip-Flop/2
  Logical Operator1/1 -> Logical Operator3/1
  Constant/1 -> D Flip-Flop/3
  D Flip-Flop/1 -> Q/1, Logical Operator2/2
  Logical Operator3/1 -> D Flip-Flop/1
  Logical Operator/1 -> Logical Operator2/1
  WE/1 -> Logical Operator/1, Logical Operator1/2
  D/1 -> Logical Operator1/1

== system Digital-Memory-Architecture/BitCell51 ==
  D : Inport
  WE : Inport  Port=2
  CLK : Inport  Port=3
  Constant : Constant
  D Flip-Flop : simulink_extras/Flip Flops/D Flip-Flop
  Logical Operator : Logic  Operator=NOT  IconShape=distinctive  AllPortsSameDT=off  OutDataTypeStr=boolean
  Logical Operator1 : Logic  IconShape=distinctive  AllPortsSameDT=off  OutDataTypeStr=boolean
  Logical Operator2 : Logic  IconShape=distinctive  AllPortsSameDT=off  OutDataTypeStr=boolean
  Logical Operator3 : Logic  Operator=OR  IconShape=distinctive  AllPortsSameDT=off  OutDataTypeStr=boolean
  Q : Outport
  wires:
  Logical Operator2/1 -> Logical Operator3/2
  CLK/1 -> D Flip-Flop/2
  Logical Operator1/1 -> Logical Operator3/1
  Constant/1 -> D Flip-Flop/3
  D Flip-Flop/1 -> Q/1, Logical Operator2/2
  Logical Operator3/1 -> D Flip-Flop/1
  Logical Operator/1 -> Logical Operator2/1
  WE/1 -> Logical Operator/1, Logical Operator1/2
  D/1 -> Logical Operator1/1

== system Digital-Memory-Architecture/BitCell52 ==
  D : Inport
  WE : Inport  Port=2
  CLK : Inport  Port=3
  Constant : Constant
  D Flip-Flop : simulink_extras/Flip Flops/D Flip-Flop
  Logical Operator : Logic  Operator=NOT  IconShape=distinctive  AllPortsSameDT=off  OutDataTypeStr=boolean
  Logical Operator1 : Logic  IconShape=distinctive  AllPortsSameDT=off  OutDataTypeStr=boolean
  Logical Operator2 : Logic  IconShape=distinctive  AllPortsSameDT=off  OutDataTypeStr=boolean
  Logical Operator3 : Logic  Operator=OR  IconShape=distinctive  AllPortsSameDT=off  OutDataTypeStr=boolean
  Q : Outport
  wires:
  Logical Operator2/1 -> Logical Operator3/2
  CLK/1 -> D Flip-Flop/2
  Logical Operator1/1 -> Logical Operator3/1
  Constant/1 -> D Flip-Flop/3
  D Flip-Flop/1 -> Q/1, Logical Operator2/2
  Logical Operator3/1 -> D Flip-Flop/1
  Logical Operator/1 -> Logical Operator2/1
  WE/1 -> Logical Operator/1, Logical Operator1/2
  D/1 -> Logical Operator1/1

== system Digital-Memory-Architecture/BitCell53 ==
  D : Inport
  WE : Inport  Port=2
  CLK : Inport  Port=3
  Constant : Constant
  D Flip-Flop : simulink_extras/Flip Flops/D Flip-Flop
  Logical Operator : Logic  Operator=NOT  IconShape=distinctive  AllPortsSameDT=off  OutDataTypeStr=boolean
  Logical Operator1 : Logic  IconShape=distinctive  AllPortsSameDT=off  OutDataTypeStr=boolean
  Logical Operator2 : Logic  IconShape=distinctive  AllPortsSameDT=off  OutDataTypeStr=boolean
  Logical Operator3 : Logic  Operator=OR  IconShape=distinctive  AllPortsSameDT=off  OutDataTypeStr=boolean
  Q : Outport
  wires:
  Logical Operator2/1 -> Logical Operator3/2
  CLK/1 -> D Flip-Flop/2
  Logical Operator1/1 -> Logical Operator3/1
  Constant/1 -> D Flip-Flop/3
  D Flip-Flop/1 -> Q/1, Logical Operator2/2
  Logical Operator3/1 -> D Flip-Flop/1
  Logical Operator/1 -> Logical Operator2/1
  WE/1 -> Logical Operator/1, Logical Operator1/2
  D/1 -> Logical Operator1/1

== system Digital-Memory-Architecture/BitCell54 ==
  D : Inport
  WE : Inport  Port=2
  CLK : Inport  Port=3
  Constant : Constant
  D Flip-Flop : simulink_extras/Flip Flops/D Flip-Flop
  Logical Operator : Logic  Operator=NOT  IconShape=distinctive  AllPortsSameDT=off  OutDataTypeStr=boolean
  Logical Operator1 : Logic  IconShape=distinctive  AllPortsSameDT=off  OutDataTypeStr=boolean
  Logical Operator2 : Logic  IconShape=distinctive  AllPortsSameDT=off  OutDataTypeStr=boolean
  Logical Operator3 : Logic  Operator=OR  IconShape=distinctive  AllPortsSameDT=off  OutDataTypeStr=boolean
  Q : Outport
  wires:
  Logical Operator2/1 -> Logical Operator3/2
  CLK/1 -> D Flip-Flop/2
  Logical Operator1/1 -> Logical Operator3/1
  Constant/1 -> D Flip-Flop/3
  D Flip-Flop/1 -> Q/1, Logical Operator2/2
  Logical Operator3/1 -> D Flip-Flop/1
  Logical Operator/1 -> Logical Operator2/1
  WE/1 -> Logical Operator/1, Logical Operator1/2
  D/1 -> Logical Operator1/1

== system Digital-Memory-Architecture/BitCell55 ==
  D : Inport
  WE : Inport  Port=2
  CLK : Inport  Port=3
  Constant : Constant
  D Flip-Flop : simulink_extras/Flip Flops/D Flip-Flop
  Logical Operator : Logic  Operator=NOT  IconShape=distinctive  AllPortsSameDT=off  OutDataTypeStr=boolean
  Logical Operator1 : Logic  IconShape=distinctive  AllPortsSameDT=off  OutDataTypeStr=boolean
  Logical Operator2 : Logic  IconShape=distinctive  AllPortsSameDT=off  OutDataTypeStr=boolean
  Logical Operator3 : Logic  Operator=OR  IconShape=distinctive  AllPortsSameDT=off  OutDataTypeStr=boolean
  Q : Outport
  wires:
  Logical Operator2/1 -> Logical Operator3/2
  CLK/1 -> D Flip-Flop/2
  Logical Operator1/1 -> Logical Operator3/1
  Constant/1 -> D Flip-Flop/3
  D Flip-Flop/1 -> Q/1, Logical Operator2/2
  Logical Operator3/1 -> D Flip-Flop/1
  Logical Operator/1 -> Logical Operator2/1
  WE/1 -> Logical Operator/1, Logical Operator1/2
  D/1 -> Logical Operator1/1

== system Digital-Memory-Architecture/BitCell56 ==
  D : Inport
  WE : Inport  Port=2
  CLK : Inport  Port=3
  Constant : Constant
  D Flip-Flop : simulink_extras/Flip Flops/D Flip-Flop
  Logical Operator : Logic  Operator=NOT  IconShape=distinctive  AllPortsSameDT=off  OutDataTypeStr=boolean
  Logical Operator1 : Logic  IconShape=distinctive  AllPortsSameDT=off  OutDataTypeStr=boolean
  Logical Operator2 : Logic  IconShape=distinctive  AllPortsSameDT=off  OutDataTypeStr=boolean
  Logical Operator3 : Logic  Operator=OR  IconShape=distinctive  AllPortsSameDT=off  OutDataTypeStr=boolean
  Q : Outport
  wires:
  Logical Operator2/1 -> Logical Operator3/2
  CLK/1 -> D Flip-Flop/2
  Logical Operator1/1 -> Logical Operator3/1
  Constant/1 -> D Flip-Flop/3
  D Flip-Flop/1 -> Q/1, Logical Operator2/2
  Logical Operator3/1 -> D Flip-Flop/1
  Logical Operator/1 -> Logical Operator2/1
  WE/1 -> Logical Operator/1, Logical Operator1/2
  D/1 -> Logical Operator1/1

== system Digital-Memory-Architecture/BitCell57 ==
  D : Inport
  WE : Inport  Port=2
  CLK : Inport  Port=3
  Constant : Constant
  D Flip-Flop : simulink_extras/Flip Flops/D Flip-Flop
  Logical Operator : Logic  Operator=NOT  IconShape=distinctive  AllPortsSameDT=off  OutDataTypeStr=boolean
  Logical Operator1 : Logic  IconShape=distinctive  AllPortsSameDT=off  OutDataTypeStr=boolean
  Logical Operator2 : Logic  IconShape=distinctive  AllPortsSameDT=off  OutDataTypeStr=boolean
  Logical Operator3 : Logic  Operator=OR  IconShape=distinctive  AllPortsSameDT=off  OutDataTypeStr=boolean
  Q : Outport
  wires:
  Logical Operator2/1 -> Logical Operator3/2
  CLK/1 -> D Flip-Flop/2
  Logical Operator1/1 -> Logical Operator3/1
  Constant/1 -> D Flip-Flop/3
  D Flip-Flop/1 -> Q/1, Logical Operator2/2
  Logical Operator3/1 -> D Flip-Flop/1
  Logical Operator/1 -> Logical Operator2/1
  WE/1 -> Logical Operator/1, Logical Operator1/2
  D/1 -> Logical Operator1/1

== system Digital-Memory-Architecture/BitCell58 ==
  D : Inport
  WE : Inport  Port=2
  CLK : Inport  Port=3
  Constant : Constant
  D Flip-Flop : simulink_extras/Flip Flops/D Flip-Flop
  Logical Operator : Logic  Operator=NOT  IconShape=distinctive  AllPortsSameDT=off  OutDataTypeStr=boolean
  Logical Operator1 : Logic  IconShape=distinctive  AllPortsSameDT=off  OutDataTypeStr=boolean
  Logical Operator2 : Logic  IconShape=distinctive  AllPortsSameDT=off  OutDataTypeStr=boolean
  Logical Operator3 : Logic  Operator=OR  IconShape=distinctive  AllPortsSameDT=off  OutDataTypeStr=boolean
  Q : Outport
  wires:
  Logical Operator2/1 -> Logical Operator3/2
  CLK/1 -> D Flip-Flop/2
  Logical Operator1/1 -> Logical Operator3/1
  Constant/1 -> D Flip-Flop/3
  D Flip-Flop/1 -> Q/1, Logical Operator2/2
  Logical Operator3/1 -> D Flip-Flop/1
  Logical Operator/1 -> Logical Operator2/1
  WE/1 -> Logical Operator/1, Logical Operator1/2
  D/1 -> Logical Operator1/1

== system Digital-Memory-Architecture/BitCell59 ==
  D : Inport
  WE : Inport  Port=2
  CLK : Inport  Port=3
  Constant : Constant
  D Flip-Flop : simulink_extras/Flip Flops/D Flip-Flop
  Logical Operator : Logic  Operator=NOT  IconShape=distinctive  AllPortsSameDT=off  OutDataTypeStr=boolean
  Logical Operator1 : Logic  IconShape=distinctive  AllPortsSameDT=off  OutDataTypeStr=boolean
  Logical Operator2 : Logic  IconShape=distinctive  AllPortsSameDT=off  OutDataTypeStr=boolean
  Logical Operator3 : Logic  Operator=OR  IconShape=distinctive  AllPortsSameDT=off  OutDataTypeStr=boolean
  Q : Outport
  wires:
  Logical Operator2/1 -> Logical Operator3/2
  CLK/1 -> D Flip-Flop/2
  Logical Operator1/1 -> Logical Operator3/1
  Constant/1 -> D Flip-Flop/3
  D Flip-Flop/1 -> Q/1, Logical Operator2/2
  Logical Operator3/1 -> D Flip-Flop/1
  Logical Operator/1 -> Logical Operator2/1
  WE/1 -> Logical Operator/1, Logical Operator1/2
  D/1 -> Logical Operator1/1

== system Digital-Memory-Architecture/BitCell6 ==
  D : Inport
  WE : Inport  Port=2
  CLK : Inport  Port=3
  Constant : Constant
  D Flip-Flop : simulink_extras/Flip Flops/D Flip-Flop
  Logical Operator : Logic  Operator=NOT  IconShape=distinctive  AllPortsSameDT=off  OutDataTypeStr=boolean
  Logical Operator1 : Logic  IconShape=distinctive  AllPortsSameDT=off  OutDataTypeStr=boolean
  Logical Operator2 : Logic  IconShape=distinctive  AllPortsSameDT=off  OutDataTypeStr=boolean
  Logical Operator3 : Logic  Operator=OR  IconShape=distinctive  AllPortsSameDT=off  OutDataTypeStr=boolean
  Q : Outport
  wires:
  Logical Operator2/1 -> Logical Operator3/2
  CLK/1 -> D Flip-Flop/2
  Logical Operator1/1 -> Logical Operator3/1
  Constant/1 -> D Flip-Flop/3
  D Flip-Flop/1 -> Q/1, Logical Operator2/2
  Logical Operator3/1 -> D Flip-Flop/1
  Logical Operator/1 -> Logical Operator2/1
  WE/1 -> Logical Operator/1, Logical Operator1/2
  D/1 -> Logical Operator1/1

== system Digital-Memory-Architecture/BitCell60 ==
  D : Inport
  WE : Inport  Port=2
  CLK : Inport  Port=3
  Constant : Constant
  D Flip-Flop : simulink_extras/Flip Flops/D Flip-Flop
  Logical Operator : Logic  Operator=NOT  IconShape=distinctive  AllPortsSameDT=off  OutDataTypeStr=boolean
  Logical Operator1 : Logic  IconShape=distinctive  AllPortsSameDT=off  OutDataTypeStr=boolean
  Logical Operator2 : Logic  IconShape=distinctive  AllPortsSameDT=off  OutDataTypeStr=boolean
  Logical Operator3 : Logic  Operator=OR  IconShape=distinctive  AllPortsSameDT=off  OutDataTypeStr=boolean
  Q : Outport
  wires:
  Logical Operator2/1 -> Logical Operator3/2
  CLK/1 -> D Flip-Flop/2
  Logical Operator1/1 -> Logical Operator3/1
  Constant/1 -> D Flip-Flop/3
  D Flip-Flop/1 -> Q/1, Logical Operator2/2
  Logical Operator3/1 -> D Flip-Flop/1
  Logical Operator/1 -> Logical Operator2/1
  WE/1 -> Logical Operator/1, Logical Operator1/2
  D/1 -> Logical Operator1/1

== system Digital-Memory-Architecture/BitCell61 ==
  D : Inport
  WE : Inport  Port=2
  CLK : Inport  Port=3
  Constant : Constant
  D Flip-Flop : simulink_extras/Flip Flops/D Flip-Flop
  Logical Operator : Logic  Operator=NOT  IconShape=distinctive  AllPortsSameDT=off  OutDataTypeStr=boolean
  Logical Operator1 : Logic  IconShape=distinctive  AllPortsSameDT=off  OutDataTypeStr=boolean
  Logical Operator2 : Logic  IconShape=distinctive  AllPortsSameDT=off  OutDataTypeStr=boolean
  Logical Operator3 : Logic  Operator=OR  IconShape=distinctive  AllPortsSameDT=off  OutDataTypeStr=boolean
  Q : Outport
  wires:
  Logical Operator2/1 -> Logical Operator3/2
  CLK/1 -> D Flip-Flop/2
  Logical Operator1/1 -> Logical Operator3/1
  Constant/1 -> D Flip-Flop/3
  D Flip-Flop/1 -> Q/1, Logical Operator2/2
  Logical Operator3/1 -> D Flip-Flop/1
  Logical Operator/1 -> Logical Operator2/1
  WE/1 -> Logical Operator/1, Logical Operator1/2
  D/1 -> Logical Operator1/1

== system Digital-Memory-Architecture/BitCell62 ==
  D : Inport
  WE : Inport  Port=2
  CLK : Inport  Port=3
  Constant : Constant
  D Flip-Flop : simulink_extras/Flip Flops/D Flip-Flop
  Logical Operator : Logic  Operator=NOT  IconShape=distinctive  AllPortsSameDT=off  OutDataTypeStr=boolean
  Logical Operator1 : Logic  IconShape=distinctive  AllPortsSameDT=off  OutDataTypeStr=boolean
  Logical Operator2 : Logic  IconShape=distinctive  AllPortsSameDT=off  OutDataTypeStr=boolean
  Logical Operator3 : Logic  Operator=OR  IconShape=distinctive  AllPortsSameDT=off  OutDataTypeStr=boolean
  Q : Outport
  wires:
  Logical Operator2/1 -> Logical Operator3/2
  CLK/1 -> D Flip-Flop/2
  Logical Operator1/1 -> Logical Operator3/1
  Constant/1 -> D Flip-Flop/3
  D Flip-Flop/1 -> Q/1, Logical Operator2/2
  Logical Operator3/1 -> D Flip-Flop/1
  Logical Operator/1 -> Logical Operator2/1
  WE/1 -> Logical Operator/1, Logical Operator1/2
  D/1 -> Logical Operator1/1

== system Digital-Memory-Architecture/BitCell63 ==
  D : Inport
  WE : Inport  Port=2
  CLK : Inport  Port=3
  Constant : Constant
  D Flip-Flop : simulink_extras/Flip Flops/D Flip-Flop
  Logical Operator : Logic  Operator=NOT  IconShape=distinctive  AllPortsSameDT=off  OutDataTypeStr=boolean
  Logical Operator1 : Logic  IconShape=distinctive  AllPortsSameDT=off  OutDataTypeStr=boolean
  Logical Operator2 : Logic  IconShape=distinctive  AllPortsSameDT=off  OutDataTypeStr=boolean
  Logical Operator3 : Logic  Operator=OR  IconShape=distinctive  AllPortsSameDT=off  OutDataTypeStr=boolean
  Q : Outport
  wires:
  Logical Operator2/1 -> Logical Operator3/2
  CLK/1 -> D Flip-Flop/2
  Logical Operator1/1 -> Logical Operator3/1
  Constant/1 -> D Flip-Flop/3
  D Flip-Flop/1 -> Q/1, Logical Operator2/2
  Logical Operator3/1 -> D Flip-Flop/1
  Logical Operator/1 -> Logical Operator2/1
  WE/1 -> Logical Operator/1, Logical Operator1/2
  D/1 -> Logical Operator1/1

== system Digital-Memory-Architecture/BitCell64 ==
  D : Inport
  WE : Inport  Port=2
  CLK : Inport  Port=3
  Constant : Constant
  D Flip-Flop : simulink_extras/Flip Flops/D Flip-Flop
  Logical Operator : Logic  Operator=NOT  IconShape=distinctive  AllPortsSameDT=off  OutDataTypeStr=boolean
  Logical Operator1 : Logic  IconShape=distinctive  AllPortsSameDT=off  OutDataTypeStr=boolean
  Logical Operator2 : Logic  IconShape=distinctive  AllPortsSameDT=off  OutDataTypeStr=boolean
  Logical Operator3 : Logic  Operator=OR  IconShape=distinctive  AllPortsSameDT=off  OutDataTypeStr=boolean
  Q : Outport
  wires:
  Logical Operator2/1 -> Logical Operator3/2
  CLK/1 -> D Flip-Flop/2
  Logical Operator1/1 -> Logical Operator3/1
  Constant/1 -> D Flip-Flop/3
  D Flip-Flop/1 -> Q/1, Logical Operator2/2
  Logical Operator3/1 -> D Flip-Flop/1
  Logical Operator/1 -> Logical Operator2/1
  WE/1 -> Logical Operator/1, Logical Operator1/2
  D/1 -> Logical Operator1/1

== system Digital-Memory-Architecture/BitCell65 ==
  D : Inport
  WE : Inport  Port=2
  CLK : Inport  Port=3
  Constant : Constant
  D Flip-Flop : simulink_extras/Flip Flops/D Flip-Flop
  Logical Operator : Logic  Operator=NOT  IconShape=distinctive  AllPortsSameDT=off  OutDataTypeStr=boolean
  Logical Operator1 : Logic  IconShape=distinctive  AllPortsSameDT=off  OutDataTypeStr=boolean
  Logical Operator2 : Logic  IconShape=distinctive  AllPortsSameDT=off  OutDataTypeStr=boolean
  Logical Operator3 : Logic  Operator=OR  IconShape=distinctive  AllPortsSameDT=off  OutDataTypeStr=boolean
  Q : Outport
  wires:
  Logical Operator2/1 -> Logical Operator3/2
  CLK/1 -> D Flip-Flop/2
  Logical Operator1/1 -> Logical Operator3/1
  Constant/1 -> D Flip-Flop/3
  D Flip-Flop/1 -> Q/1, Logical Operator2/2
  Logical Operator3/1 -> D Flip-Flop/1
  Logical Operator/1 -> Logical Operator2/1
  WE/1 -> Logical Operator/1, Logical Operator1/2
  D/1 -> Logical Operator1/1

== system Digital-Memory-Architecture/BitCell66 ==
  D : Inport
  WE : Inport  Port=2
  CLK : Inport  Port=3
  Constant : Constant
  D Flip-Flop : simulink_extras/Flip Flops/D Flip-Flop
  Logical Operator : Logic  Operator=NOT  IconShape=distinctive  AllPortsSameDT=off  OutDataTypeStr=boolean
  Logical Operator1 : Logic  IconShape=distinctive  AllPortsSameDT=off  OutDataTypeStr=boolean
  Logical Operator2 : Logic  IconShape=distinctive  AllPortsSameDT=off  OutDataTypeStr=boolean
  Logical Operator3 : Logic  Operator=OR  IconShape=distinctive  AllPortsSameDT=off  OutDataTypeStr=boolean
  Q : Outport
  wires:
  Logical Operator2/1 -> Logical Operator3/2
  CLK/1 -> D Flip-Flop/2
  Logical Operator1/1 -> Logical Operator3/1
  Constant/1 -> D Flip-Flop/3
  D Flip-Flop/1 -> Q/1, Logical Operator2/2
  Logical Operator3/1 -> D Flip-Flop/1
  Logical Operator/1 -> Logical Operator2/1
  WE/1 -> Logical Operator/1, Logical Operator1/2
  D/1 -> Logical Operator1/1

== system Digital-Memory-Architecture/BitCell67 ==
  D : Inport
  WE : Inport  Port=2
  CLK : Inport  Port=3
  Constant : Constant
  D Flip-Flop : simulink_extras/Flip Flops/D Flip-Flop
  Logical Operator : Logic  Operator=NOT  IconShape=distinctive  AllPortsSameDT=off  OutDataTypeStr=boolean
  Logical Operator1 : Logic  IconShape=distinctive  AllPortsSameDT=off  OutDataTypeStr=boolean
  Logical Operator2 : Logic  IconShape=distinctive  AllPortsSameDT=off  OutDataTypeStr=boolean
  Logical Operator3 : Logic  Operator=OR  IconShape=distinctive  AllPortsSameDT=off  OutDataTypeStr=boolean
  Q : Outport
  wires:
  Logical Operator2/1 -> Logical Operator3/2
  CLK/1 -> D Flip-Flop/2
  Logical Operator1/1 -> Logical Operator3/1
  Constant/1 -> D Flip-Flop/3
  D Flip-Flop/1 -> Q/1, Logical Operator2/2
  Logical Operator3/1 -> D Flip-Flop/1
  Logical Operator/1 -> Logical Operator2/1
  WE/1 -> Logical Operator/1, Logical Operator1/2
  D/1 -> Logical Operator1/1

== system Digital-Memory-Architecture/BitCell68 ==
  D : Inport
  WE : Inport  Port=2
  CLK : Inport  Port=3
  Constant : Constant
  D Flip-Flop : simulink_extras/Flip Flops/D Flip-Flop
  Logical Operator : Logic  Operator=NOT  IconShape=distinctive  AllPortsSameDT=off  OutDataTypeStr=boolean
  Logical Operator1 : Logic  IconShape=distinctive  AllPortsSameDT=off  OutDataTypeStr=boolean
  Logical Operator2 : Logic  IconShape=distinctive  AllPortsSameDT=off  OutDataTypeStr=boolean
  Logical Operator3 : Logic  Operator=OR  IconShape=distinctive  AllPortsSameDT=off  OutDataTypeStr=boolean
  Q : Outport
  wires:
  Logical Operator2/1 -> Logical Operator3/2
  CLK/1 -> D Flip-Flop/2
  Logical Operator1/1 -> Logical Operator3/1
  Constant/1 -> D Flip-Flop/3
  D Flip-Flop/1 -> Q/1, Logical Operator2/2
  Logical Operator3/1 -> D Flip-Flop/1
  Logical Operator/1 -> Logical Operator2/1
  WE/1 -> Logical Operator/1, Logical Operator1/2
  D/1 -> Logical Operator1/1

== system Digital-Memory-Architecture/BitCell69 ==
  D : Inport
  WE : Inport  Port=2
  CLK : Inport  Port=3
  Constant : Constant
  D Flip-Flop : simulink_extras/Flip Flops/D Flip-Flop
  Logical Operator : Logic  Operator=NOT  IconShape=distinctive  AllPortsSameDT=off  OutDataTypeStr=boolean
  Logical Operator1 : Logic  IconShape=distinctive  AllPortsSameDT=off  OutDataTypeStr=boolean
  Logical Operator2 : Logic  IconShape=distinctive  AllPortsSameDT=off  OutDataTypeStr=boolean
  Logical Operator3 : Logic  Operator=OR  IconShape=distinctive  AllPortsSameDT=off  OutDataTypeStr=boolean
  Q : Outport
  wires:
  Logical Operator2/1 -> Logical Operator3/2
  CLK/1 -> D Flip-Flop/2
  Logical Operator1/1 -> Logical Operator3/1
  Constant/1 -> D Flip-Flop/3
  D Flip-Flop/1 -> Q/1, Logical Operator2/2
  Logical Operator3/1 -> D Flip-Flop/1
  Logical Operator/1 -> Logical Operator2/1
  WE/1 -> Logical Operator/1, Logical Operator1/2
  D/1 -> Logical Operator1/1
